simulink model "ThermalTank_ClosedLoop_Reference"  (R2023a)
settings: Solver=ode4  StartTime=0.0  StopTime=8  FixedStep=0.001  RelTol=1e-3
settings Model: Creator=Fasih  LastModifiedBy=Fasih

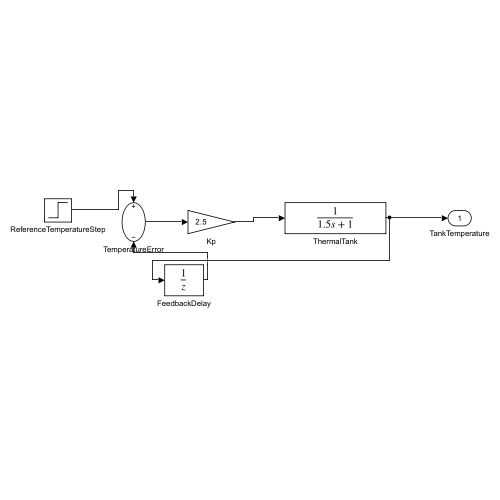
[thumbnail: Simulink's stored preview of the top-level diagram]
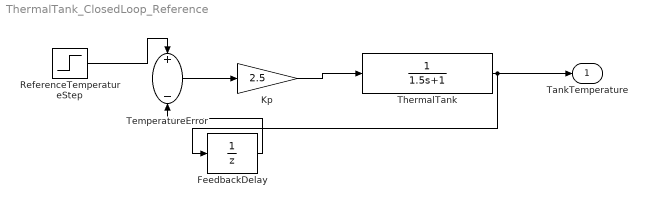
== system ThermalTank_ClosedLoop_Reference ==
  FeedbackDelay : UnitDelay  SampleTime=0.001  HasFrameUpgradeWarning=on
  Kp : Gain  Gain=2.5
  ReferenceTemperatureStep : Step  Time=0  SampleTime=0
  TemperatureError : Sum  Inputs=+-
  ThermalTank : TransferFcn  Denominator=[1.5 1]
  TankTemperature : Outport
  wires:
  ReferenceTemperatureStep/1 -> TemperatureError/1
  FeedbackDelay/1 -> TemperatureError/2
  TemperatureError/1 -> Kp/1
  Kp/1 -> ThermalTank/1
  ThermalTank/1 -> TankTemperature/1, FeedbackDelay/1
